simulink model "temp"  (R2013b)
settings: Solver=ode45  StartTime=0.0  StopTime=100*100  RelTol=1e-3
undefined symbols (not defined in the file or in its folder): gray
libraries: xbsIndex_r4 x52, dspsigattribs x9, visionsinks x3, visionsources x1
settings Model: Creator=Sechw  LastModifiedBy=Sechw

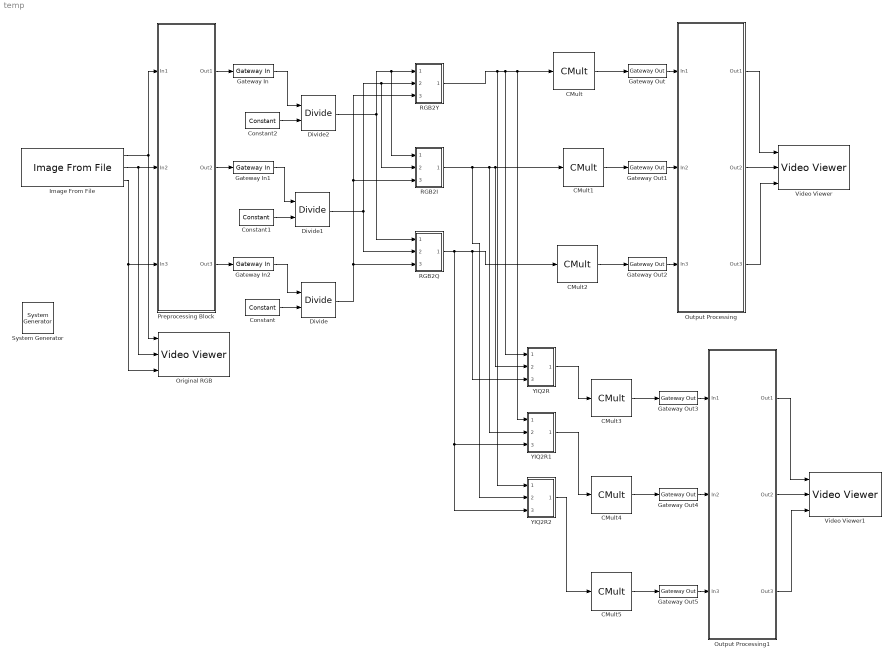
== system temp ==
  " System Generator" : xbsIndex_r4/ System Generator  Tag=genX  xilinxfamily=virtex6  part=xc6vlx130t  speed=-1  package=ff1156  synthesis_tool=XST  clock_wrapper=Clock Enables  directory=./netlist  proj_type=Project Navigator  Synth_file=XST Defaults  Impl_file=ISE Defaults  testbench=off  simulink_period=1  sysclk_period=10  dcm_input_clock_period=10  incr_netlist=off  trim_vbits=Everywhere in SubSystem  dbl_ovrd=According to Block Masks  core_generation=According to Block Masks  run_coregen=off  deprecated_control=off  eval_field=0  block_type=sysgen
  CMult{,1..5} (6 alike) : xbsIndex_r4/CMult  const=255  gui_display_data_type=Floating-point  const_n_bits=16  const_bin_pt=14  float_type=Double  exp_bits=8  fraction_bits=24  en=off  latency=0  precision=Full  arith_type="Signed  (2's comp)"  n_bits=16  bin_pt=14  quantization=Truncate  overflow=Wrap  dbl_ovrd=off  use_behavioral_HDL=off  mem_type=Distributed RAM  pipeline=off  block_type=cmult
  Constant : xbsIndex_r4/Constant  const=255  gui_display_data_type=Floating-point  arith_type=Floating-point  n_bits=16  bin_pt=14  preci_type=Double  exp_width=8  frac_width=24  explicit_period=off  period=1  equ=P=C  opselect=C  inp2=PCIN>>17  opr=+  inp1=P  carry=CIN  dbl_ovrd=off  block_type=constant
  Constant1 : xbsIndex_r4/Constant  const=255  gui_display_data_type=Floating-point  arith_type=Floating-point  n_bits=16  bin_pt=14  preci_type=Double  exp_width=8  frac_width=24  explicit_period=off  period=1  equ=P=C  opselect=C  inp2=PCIN>>17  opr=+  inp1=P  carry=CIN  dbl_ovrd=off  block_type=constant
  Constant2 : xbsIndex_r4/Constant  const=255  gui_display_data_type=Floating-point  arith_type=Floating-point  n_bits=16  bin_pt=14  preci_type=Double  exp_width=8  frac_width=24  explicit_period=off  period=1  equ=P=C  opselect=C  inp2=PCIN>>17  opr=+  inp1=P  carry=CIN  dbl_ovrd=off  block_type=constant
  Divide : xbsIndex_r4/Divide  flow_control=NonBlocking  axi_optimize_goal=Resources  algorithm_type=High_Radix  infoedit1=Specify output fraction-width for Fixed-point division.  fractional_width=16  latency=0  rate=1  has_a_tlast=off  has_a_tuser=off  has_b_tlast=off  has_b_tuser=off  en=off  has_result_tready=off  result_tlast_behv=Pass_A_TLAST  has_underflow=off  has_overflow=off  has_invalid_op=off  has_divide_by_zero=off  fpo_op_type=mergeddivide  block_type=divide
      settings: infoedit=Blocking: Wait for data on all inputs, allow back-pressure.<br>NonBlocking: operate every cycle in which all inputs are valid, no back-pressure.
  Divide1 : xbsIndex_r4/Divide  flow_control=NonBlocking  axi_optimize_goal=Resources  algorithm_type=High_Radix  infoedit1=Specify output fraction-width for Fixed-point division.  fractional_width=16  latency=0  rate=1  has_a_tlast=off  has_a_tuser=off  has_b_tlast=off  has_b_tuser=off  en=off  has_result_tready=off  result_tlast_behv=Pass_A_TLAST  has_underflow=off  has_overflow=off  has_invalid_op=off  has_divide_by_zero=off  fpo_op_type=mergeddivide  block_type=divide
      settings: infoedit=Blocking: Wait for data on all inputs, allow back-pressure.<br>NonBlocking: operate every cycle in which all inputs are valid, no back-pressure.
  Divide2 : xbsIndex_r4/Divide  flow_control=NonBlocking  axi_optimize_goal=Resources  algorithm_type=High_Radix  infoedit1=Specify output fraction-width for Fixed-point division.  fractional_width=16  latency=0  rate=1  has_a_tlast=off  has_a_tuser=off  has_b_tlast=off  has_b_tuser=off  en=off  has_result_tready=off  result_tlast_behv=Pass_A_TLAST  has_underflow=off  has_overflow=off  has_invalid_op=off  has_divide_by_zero=off  fpo_op_type=mergeddivide  block_type=divide
      settings: infoedit=Blocking: Wait for data on all inputs, allow back-pressure.<br>NonBlocking: operate every cycle in which all inputs are valid, no back-pressure.
  Gateway In : xbsIndex_r4/Gateway In  gui_display_data_type=Floating-point  arith_type=Floating-point  n_bits=8  bin_pt=0  preci_type=Double  exp_width=8  frac_width=24  quantization="Round  (unbiased: +/- Inf)"  overflow=Saturate  period=1  dbl_ovrd=off  timing_constraint=None  locs_specified=off  LOCs={}  UseAsADC=off  ADCChannel='1'  inherit_from_input=off  hdl_port=on  block_type=gatewayin
  Gateway In1 : xbsIndex_r4/Gateway In  gui_display_data_type=Floating-point  arith_type=Floating-point  n_bits=8  bin_pt=0  preci_type=Double  exp_width=8  frac_width=24  quantization="Round  (unbiased: +/- Inf)"  overflow=Saturate  period=1  dbl_ovrd=off  timing_constraint=None  locs_specified=off  LOCs={}  UseAsADC=off  ADCChannel='1'  inherit_from_input=off  hdl_port=on  block_type=gatewayin
  Gateway In2 : xbsIndex_r4/Gateway In  gui_display_data_type=Floating-point  arith_type=Floating-point  n_bits=8  bin_pt=0  preci_type=Double  exp_width=8  frac_width=24  quantization="Round  (unbiased: +/- Inf)"  overflow=Saturate  period=1  dbl_ovrd=off  timing_constraint=None  locs_specified=off  LOCs={}  UseAsADC=off  ADCChannel='1'  inherit_from_input=off  hdl_port=on  block_type=gatewayin
  Gateway Out{,1..5} (6 alike) : xbsIndex_r4/Gateway Out  inherit_from_input=on  hdl_port=on  timing_constraint=None  locs_specified=off  LOCs={}  UseAsDAC=off  DACChannel='1'  block_type=gatewayout
  Image From File : visionsources/Image From File  Tag=vipblks_nd  FileName=C:\Users\Sechw\Documents\MATLAB\4440\lena.jpg  imagePorts=Separate color signals  Ts=inf  ImageDataType=Inherit from input image  Signed=on  WordLength=16  sdImageDataType=uint(8)  FractionLengthMode=User-defined  FractionLength=15  OutPortLabels=R|G|B
  Original RGB : visionsinks/Video Viewer  inputType=Obsolete7b  imagePorts=Separate color signals  useColorMap=off  colormapValue=gray(256)  specRange=off  minInputVal=0  maxInputVal=255  FigPos=[692 476 183 243]  AxisZoom=on  trueSizedOnce=off  OpenAtMdlStart=on  DefaultConfigurationName=vipscopes.VideoViewerScopeCfg
  Output Processing : Subsystem
  Output Processing1 : Subsystem
  Preprocessing Block : Subsystem
  RGB2I : Subsystem
  RGB2Q : Subsystem
  RGB2Y : Subsystem
  Video Viewer : visionsinks/Video Viewer  inputType=Obsolete7b  imagePorts=Separate color signals  useColorMap=off  colormapValue=gray(256)  specRange=off  minInputVal=0  maxInputVal=255  FigPos=[437 462 320 274]  AxisZoom=on  trueSizedOnce=off  OpenAtMdlStart=on  DefaultConfigurationName=vipscopes.VideoViewerScopeCfg
  Video Viewer1 : visionsinks/Video Viewer  inputType=Obsolete7b  imagePorts=Separate color signals  useColorMap=off  colormapValue=gray(256)  specRange=off  minInputVal=0  maxInputVal=255  FigPos=[775 461 441 293]  AxisZoom=on  trueSizedOnce=off  OpenAtMdlStart=on  DefaultConfigurationName=vipscopes.VideoViewerScopeCfg
  YIQ2R : Subsystem
  YIQ2R1 : Subsystem
  YIQ2R2 : Subsystem
  wires:
  Image From File/1 -> Preprocessing Block/1(In1), Original RGB/1
  Image From File/2 -> Original RGB/2, Preprocessing Block/2(In2)
  Image From File/3 -> Original RGB/3, Preprocessing Block/3(In3)
  Preprocessing Block/1(Out1) -> Gateway In/1
  Preprocessing Block/2(Out2) -> Gateway In1/1
  Preprocessing Block/3(Out3) -> Gateway In2/1
  Gateway Out/1 -> Output Processing/1(In1)
  Gateway Out1/1 -> Output Processing/2(In2)
  Gateway Out2/1 -> Output Processing/3(In3)
  Output Processing/1(Out1) -> Video Viewer/1
  Output Processing/2(Out2) -> Video Viewer/2
  Output Processing/3(Out3) -> Video Viewer/3
  Divide2/1 -> RGB2I/1(In1), RGB2Y/1(In1), RGB2Q/1(In1)
  Divide1/1 -> RGB2I/2(In2), RGB2Y/2(In2), RGB2Q/2(In2)
  Divide/1 -> RGB2Q/3(In3), RGB2Y/3(In3), RGB2I/3(In3)
  RGB2Y/1(Out1) -> YIQ2R2/1(In1), YIQ2R/1(In1), YIQ2R1/1(In1), CMult/1
  RGB2I/1(Out1) -> YIQ2R2/2(In2), YIQ2R1/2(In2), YIQ2R/2(In2), CMult1/1
  RGB2Q/1(Out1) -> YIQ2R2/3(In3), YIQ2R1/3(In3), YIQ2R/3(In3), CMult2/1
  Gateway Out3/1 -> Output Processing1/1(In1)
  Gateway Out4/1 -> Output Processing1/2(In2)
  Gateway Out5/1 -> Output Processing1/3(In3)
  Output Processing1/1(Out1) -> Video Viewer1/1
  Output Processing1/2(Out2) -> Video Viewer1/2
  Output Processing1/3(Out3) -> Video Viewer1/3
  YIQ2R/1(Out1) -> CMult3/1
  YIQ2R1/1(Out1) -> CMult4/1
  YIQ2R2/1(Out1) -> CMult5/1
  Gateway In2/1 -> Divide/1
  Constant/1 -> Divide/2
  CMult/1 -> Gateway Out/1
  CMult1/1 -> Gateway Out1/1
  CMult2/1 -> Gateway Out2/1
  Gateway In1/1 -> Divide1/1
  Constant1/1 -> Divide1/2
  Gateway In/1 -> Divide2/1
  Constant2/1 -> Divide2/2
  CMult3/1 -> Gateway Out3/1
  CMult4/1 -> Gateway Out4/1
  CMult5/1 -> Gateway Out5/1

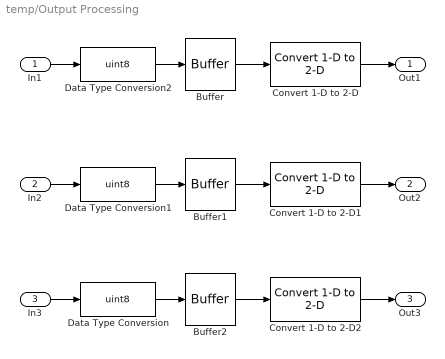
== system temp/Output Processing ==
  In1 : Inport
  In2 : Inport  Port=2
  In3 : Inport  Port=3
  Buffer : Buffer  N=100*100  TreatMby1Signals=One channel
  Buffer1 : Buffer  N=100*100  TreatMby1Signals=One channel
  Buffer2 : Buffer  N=100*100  TreatMby1Signals=One channel
  Convert 1-D to 2-D : dspsigattribs/Convert 1-D to 2-D  M=100  N=100  frameBasedOut=off
  Convert 1-D to 2-D1 : dspsigattribs/Convert 1-D to 2-D  M=100  N=100  frameBasedOut=off
  Convert 1-D to 2-D2 : dspsigattribs/Convert 1-D to 2-D  M=100  N=100  frameBasedOut=off
  Data Type Conversion : DataTypeConversion  OutDataTypeStr=uint8
  Data Type Conversion1 : DataTypeConversion  OutDataTypeStr=uint8
  Data Type Conversion2 : DataTypeConversion  OutDataTypeStr=uint8
  Out1 : Outport
  Out2 : Outport  Port=2
  Out3 : Outport  Port=3
  wires:
  Convert 1-D to 2-D2/1 -> Out3/1
  Convert 1-D to 2-D1/1 -> Out2/1
  Buffer1/1 -> Convert 1-D to 2-D1/1
  Buffer2/1 -> Convert 1-D to 2-D2/1
  Buffer/1 -> Convert 1-D to 2-D/1
  Convert 1-D to 2-D/1 -> Out1/1
  In1/1 -> Data Type Conversion2/1
  In2/1 -> Data Type Conversion1/1
  In3/1 -> Data Type Conversion/1
  Data Type Conversion/1 -> Buffer2/1
  Data Type Conversion1/1 -> Buffer1/1
  Data Type Conversion2/1 -> Buffer/1

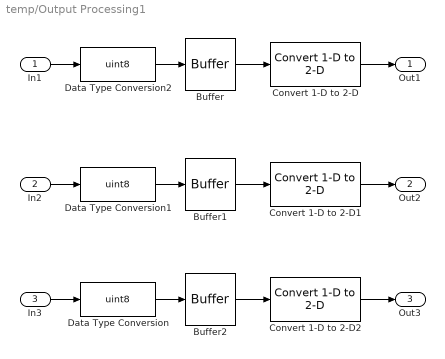
== system temp/Output Processing1 ==
  In1 : Inport
  In2 : Inport  Port=2
  In3 : Inport  Port=3
  Buffer : Buffer  N=100*100  TreatMby1Signals=One channel
  Buffer1 : Buffer  N=100*100  TreatMby1Signals=One channel
  Buffer2 : Buffer  N=100*100  TreatMby1Signals=One channel
  Convert 1-D to 2-D : dspsigattribs/Convert 1-D to 2-D  M=100  N=100  frameBasedOut=off
  Convert 1-D to 2-D1 : dspsigattribs/Convert 1-D to 2-D  M=100  N=100  frameBasedOut=off
  Convert 1-D to 2-D2 : dspsigattribs/Convert 1-D to 2-D  M=100  N=100  frameBasedOut=off
  Data Type Conversion : DataTypeConversion  OutDataTypeStr=uint8
  Data Type Conversion1 : DataTypeConversion  OutDataTypeStr=uint8
  Data Type Conversion2 : DataTypeConversion  OutDataTypeStr=uint8
  Out1 : Outport
  Out2 : Outport  Port=2
  Out3 : Outport  Port=3
  wires:
  Convert 1-D to 2-D2/1 -> Out3/1
  Convert 1-D to 2-D1/1 -> Out2/1
  Buffer1/1 -> Convert 1-D to 2-D1/1
  Buffer2/1 -> Convert 1-D to 2-D2/1
  Buffer/1 -> Convert 1-D to 2-D/1
  Convert 1-D to 2-D/1 -> Out1/1
  In1/1 -> Data Type Conversion2/1
  In2/1 -> Data Type Conversion1/1
  In3/1 -> Data Type Conversion/1
  Data Type Conversion/1 -> Buffer2/1
  Data Type Conversion1/1 -> Buffer1/1
  Data Type Conversion2/1 -> Buffer/1

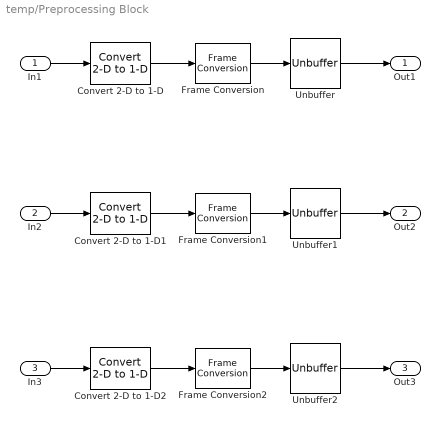
== system temp/Preprocessing Block ==
  In1 : Inport
  In2 : Inport  Port=2
  In3 : Inport  Port=3
  Convert 2-D to 1-D : dspsigattribs/Convert 2-D to 1-D
  Convert 2-D to 1-D1 : dspsigattribs/Convert 2-D to 1-D
  Convert 2-D to 1-D2 : dspsigattribs/Convert 2-D to 1-D
  Frame Conversion : FrameConversion
  Frame Conversion1 : FrameConversion
  Frame Conversion2 : FrameConversion
  Unbuffer : Unbuffer  SampleBasedProcessing=Same as frame based
  Unbuffer1 : Unbuffer  SampleBasedProcessing=Same as frame based
  Unbuffer2 : Unbuffer  SampleBasedProcessing=Same as frame based
  Out1 : Outport
  Out2 : Outport  Port=2
  Out3 : Outport  Port=3
  wires:
  In1/1 -> Convert 2-D to 1-D/1
  Frame Conversion1/1 -> Unbuffer1/1
  Convert 2-D to 1-D1/1 -> Frame Conversion1/1
  In2/1 -> Convert 2-D to 1-D1/1
  Unbuffer1/1 -> Out2/1
  Frame Conversion2/1 -> Unbuffer2/1
  In3/1 -> Convert 2-D to 1-D2/1
  Convert 2-D to 1-D2/1 -> Frame Conversion2/1
  Unbuffer2/1 -> Out3/1
  Unbuffer/1 -> Out1/1
  Frame Conversion/1 -> Unbuffer/1
  Convert 2-D to 1-D/1 -> Frame Conversion/1

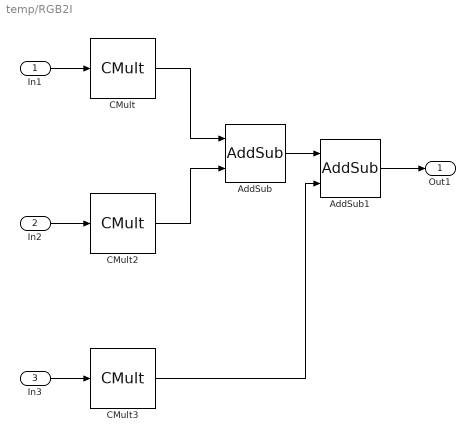
== system temp/RGB2I ==
  In1 : Inport
  In2 : Inport  Port=2
  In3 : Inport  Port=3
  AddSub : xbsIndex_r4/AddSub  mode=Addition  use_carryin=off  use_carryout=off  en=off  latency=0  precision=Full  arith_type=Unsigned  n_bits=16  bin_pt=14  quantization=Truncate  overflow=Wrap  dbl_ovrd=off  use_behavioral_HDL=off  hw_selection=Fabric  pipelined=off  block_type=addsub
  AddSub1 : xbsIndex_r4/AddSub  mode=Addition  use_carryin=off  use_carryout=off  en=off  latency=0  precision=Full  arith_type=Unsigned  n_bits=16  bin_pt=14  quantization=Truncate  overflow=Wrap  dbl_ovrd=off  use_behavioral_HDL=off  hw_selection=Fabric  pipelined=off  block_type=addsub
  CMult : xbsIndex_r4/CMult  const=0.596  gui_display_data_type=Floating-point  const_n_bits=8  const_bin_pt=8  float_type=Double  exp_bits=8  fraction_bits=24  en=off  latency=0  precision=Full  arith_type="Signed  (2's comp)"  n_bits=16  bin_pt=14  quantization=Truncate  overflow=Wrap  dbl_ovrd=off  use_behavioral_HDL=off  mem_type=Distributed RAM  pipeline=off  block_type=cmult
  CMult2 : xbsIndex_r4/CMult  const=-0.275  gui_display_data_type=Floating-point  const_n_bits=8  const_bin_pt=8  float_type=Double  exp_bits=8  fraction_bits=24  en=off  latency=0  precision=Full  arith_type="Signed  (2's comp)"  n_bits=16  bin_pt=14  quantization=Truncate  overflow=Wrap  dbl_ovrd=off  use_behavioral_HDL=off  mem_type=Distributed RAM  pipeline=off  block_type=cmult
  CMult3 : xbsIndex_r4/CMult  const=-0.321  gui_display_data_type=Floating-point  const_n_bits=8  const_bin_pt=8  float_type=Double  exp_bits=8  fraction_bits=24  en=off  latency=0  precision=Full  arith_type="Signed  (2's comp)"  n_bits=16  bin_pt=14  quantization=Truncate  overflow=Wrap  dbl_ovrd=off  use_behavioral_HDL=off  mem_type=Distributed RAM  pipeline=off  block_type=cmult
  Out1 : Outport
  wires:
  In2/1 -> CMult2/1
  CMult2/1 -> AddSub/2
  AddSub/1 -> AddSub1/1
  AddSub1/1 -> Out1/1
  CMult3/1 -> AddSub1/2
  CMult/1 -> AddSub/1
  In3/1 -> CMult3/1
  In1/1 -> CMult/1

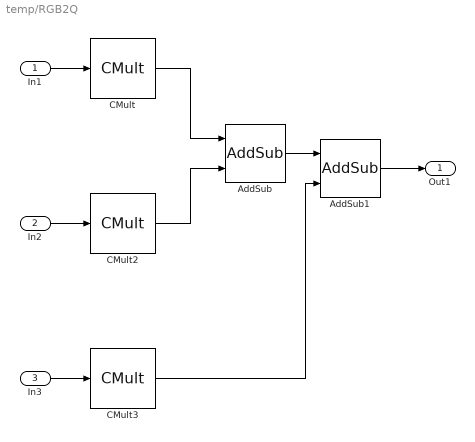
== system temp/RGB2Q ==
  In1 : Inport
  In2 : Inport  Port=2
  In3 : Inport  Port=3
  AddSub : xbsIndex_r4/AddSub  mode=Addition  use_carryin=off  use_carryout=off  en=off  latency=0  precision=Full  arith_type=Unsigned  n_bits=16  bin_pt=14  quantization=Truncate  overflow=Wrap  dbl_ovrd=off  use_behavioral_HDL=off  hw_selection=Fabric  pipelined=off  block_type=addsub
  AddSub1 : xbsIndex_r4/AddSub  mode=Addition  use_carryin=off  use_carryout=off  en=off  latency=0  precision=Full  arith_type=Unsigned  n_bits=16  bin_pt=14  quantization=Truncate  overflow=Wrap  dbl_ovrd=off  use_behavioral_HDL=off  hw_selection=Fabric  pipelined=off  block_type=addsub
  CMult : xbsIndex_r4/CMult  const=0.212  gui_display_data_type=Floating-point  const_n_bits=8  const_bin_pt=8  float_type=Double  exp_bits=8  fraction_bits=24  en=off  latency=0  precision=Full  arith_type="Signed  (2's comp)"  n_bits=16  bin_pt=14  quantization=Truncate  overflow=Wrap  dbl_ovrd=off  use_behavioral_HDL=off  mem_type=Distributed RAM  pipeline=off  block_type=cmult
  CMult2 : xbsIndex_r4/CMult  const=-0.523  gui_display_data_type=Floating-point  const_n_bits=8  const_bin_pt=8  float_type=Double  exp_bits=8  fraction_bits=24  en=off  latency=0  precision=Full  arith_type="Signed  (2's comp)"  n_bits=16  bin_pt=14  quantization=Truncate  overflow=Wrap  dbl_ovrd=off  use_behavioral_HDL=off  mem_type=Distributed RAM  pipeline=off  block_type=cmult
  CMult3 : xbsIndex_r4/CMult  const=0.311  gui_display_data_type=Floating-point  const_n_bits=8  const_bin_pt=8  float_type=Double  exp_bits=8  fraction_bits=24  en=off  latency=0  precision=Full  arith_type="Signed  (2's comp)"  n_bits=16  bin_pt=14  quantization=Truncate  overflow=Wrap  dbl_ovrd=off  use_behavioral_HDL=off  mem_type=Distributed RAM  pipeline=off  block_type=cmult
  Out1 : Outport
  wires:
  In2/1 -> CMult2/1
  CMult2/1 -> AddSub/2
  AddSub/1 -> AddSub1/1
  AddSub1/1 -> Out1/1
  CMult3/1 -> AddSub1/2
  CMult/1 -> AddSub/1
  In3/1 -> CMult3/1
  In1/1 -> CMult/1

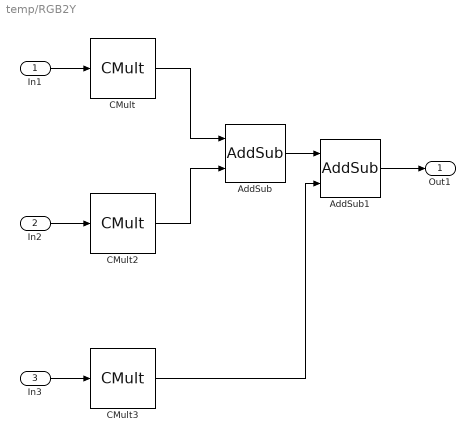
== system temp/RGB2Y ==
  In1 : Inport
  In2 : Inport  Port=2
  In3 : Inport  Port=3
  AddSub : xbsIndex_r4/AddSub  mode=Addition  use_carryin=off  use_carryout=off  en=off  latency=0  precision=Full  arith_type=Unsigned  n_bits=16  bin_pt=14  quantization=Truncate  overflow=Wrap  dbl_ovrd=off  use_behavioral_HDL=off  hw_selection=Fabric  pipelined=off  block_type=addsub
  AddSub1 : xbsIndex_r4/AddSub  mode=Addition  use_carryin=off  use_carryout=off  en=off  latency=0  precision=Full  arith_type=Unsigned  n_bits=16  bin_pt=14  quantization=Truncate  overflow=Wrap  dbl_ovrd=off  use_behavioral_HDL=off  hw_selection=Fabric  pipelined=off  block_type=addsub
  CMult : xbsIndex_r4/CMult  const=0.299  gui_display_data_type=Floating-point  const_n_bits=8  const_bin_pt=8  float_type=Double  exp_bits=8  fraction_bits=24  en=off  latency=0  precision=Full  arith_type="Signed  (2's comp)"  n_bits=16  bin_pt=14  quantization=Truncate  overflow=Wrap  dbl_ovrd=off  use_behavioral_HDL=off  mem_type=Distributed RAM  pipeline=off  block_type=cmult
  CMult2 : xbsIndex_r4/CMult  const=0.587  gui_display_data_type=Floating-point  const_n_bits=8  const_bin_pt=8  float_type=Double  exp_bits=8  fraction_bits=24  en=off  latency=0  precision=Full  arith_type="Signed  (2's comp)"  n_bits=16  bin_pt=14  quantization=Truncate  overflow=Wrap  dbl_ovrd=off  use_behavioral_HDL=off  mem_type=Distributed RAM  pipeline=off  block_type=cmult
  CMult3 : xbsIndex_r4/CMult  const=0.114  gui_display_data_type=Floating-point  const_n_bits=8  const_bin_pt=8  float_type=Double  exp_bits=8  fraction_bits=24  en=off  latency=0  precision=Full  arith_type="Signed  (2's comp)"  n_bits=16  bin_pt=14  quantization=Truncate  overflow=Wrap  dbl_ovrd=off  use_behavioral_HDL=off  mem_type=Distributed RAM  pipeline=off  block_type=cmult
  Out1 : Outport
  wires:
  In2/1 -> CMult2/1
  CMult2/1 -> AddSub/2
  AddSub/1 -> AddSub1/1
  AddSub1/1 -> Out1/1
  CMult3/1 -> AddSub1/2
  CMult/1 -> AddSub/1
  In3/1 -> CMult3/1
  In1/1 -> CMult/1

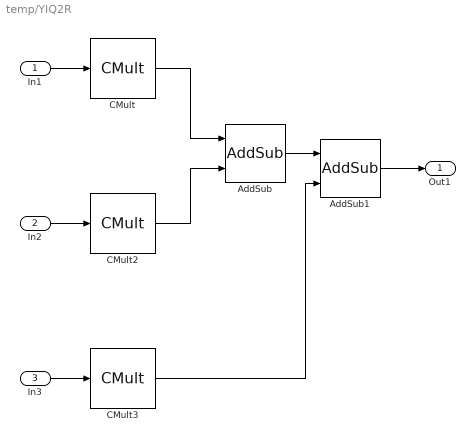
== system temp/YIQ2R ==
  In1 : Inport
  In2 : Inport  Port=2
  In3 : Inport  Port=3
  AddSub : xbsIndex_r4/AddSub  mode=Addition  use_carryin=off  use_carryout=off  en=off  latency=0  precision=Full  arith_type=Unsigned  n_bits=16  bin_pt=14  quantization=Truncate  overflow=Wrap  dbl_ovrd=off  use_behavioral_HDL=off  hw_selection=Fabric  pipelined=off  block_type=addsub
  AddSub1 : xbsIndex_r4/AddSub  mode=Addition  use_carryin=off  use_carryout=off  en=off  latency=0  precision=Full  arith_type=Unsigned  n_bits=16  bin_pt=14  quantization=Truncate  overflow=Wrap  dbl_ovrd=off  use_behavioral_HDL=off  hw_selection=Fabric  pipelined=off  block_type=addsub
  CMult : xbsIndex_r4/CMult  const=1  gui_display_data_type=Floating-point  const_n_bits=8  const_bin_pt=8  float_type=Double  exp_bits=8  fraction_bits=24  en=off  latency=0  precision=Full  arith_type="Signed  (2's comp)"  n_bits=16  bin_pt=14  quantization=Truncate  overflow=Wrap  dbl_ovrd=off  use_behavioral_HDL=off  mem_type=Distributed RAM  pipeline=off  block_type=cmult
  CMult2 : xbsIndex_r4/CMult  const=0.965  gui_display_data_type=Floating-point  const_n_bits=8  const_bin_pt=8  float_type=Double  exp_bits=8  fraction_bits=24  en=off  latency=0  precision=Full  arith_type="Signed  (2's comp)"  n_bits=16  bin_pt=14  quantization=Truncate  overflow=Wrap  dbl_ovrd=off  use_behavioral_HDL=off  mem_type=Distributed RAM  pipeline=off  block_type=cmult
  CMult3 : xbsIndex_r4/CMult  const=0.621  gui_display_data_type=Floating-point  const_n_bits=8  const_bin_pt=8  float_type=Double  exp_bits=8  fraction_bits=24  en=off  latency=0  precision=Full  arith_type="Signed  (2's comp)"  n_bits=16  bin_pt=14  quantization=Truncate  overflow=Wrap  dbl_ovrd=off  use_behavioral_HDL=off  mem_type=Distributed RAM  pipeline=off  block_type=cmult
  Out1 : Outport
  wires:
  In2/1 -> CMult2/1
  CMult2/1 -> AddSub/2
  AddSub/1 -> AddSub1/1
  AddSub1/1 -> Out1/1
  CMult3/1 -> AddSub1/2
  CMult/1 -> AddSub/1
  In3/1 -> CMult3/1
  In1/1 -> CMult/1

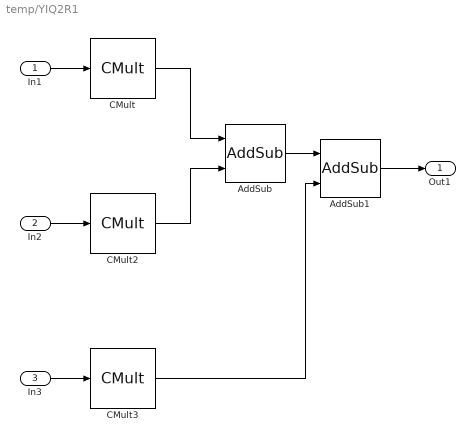
== system temp/YIQ2R1 ==
  In1 : Inport
  In2 : Inport  Port=2
  In3 : Inport  Port=3
  AddSub : xbsIndex_r4/AddSub  mode=Addition  use_carryin=off  use_carryout=off  en=off  latency=0  precision=Full  arith_type=Unsigned  n_bits=16  bin_pt=14  quantization=Truncate  overflow=Wrap  dbl_ovrd=off  use_behavioral_HDL=off  hw_selection=Fabric  pipelined=off  block_type=addsub
  AddSub1 : xbsIndex_r4/AddSub  mode=Addition  use_carryin=off  use_carryout=off  en=off  latency=0  precision=Full  arith_type=Unsigned  n_bits=16  bin_pt=14  quantization=Truncate  overflow=Wrap  dbl_ovrd=off  use_behavioral_HDL=off  hw_selection=Fabric  pipelined=off  block_type=addsub
  CMult : xbsIndex_r4/CMult  const=1  gui_display_data_type=Floating-point  const_n_bits=8  const_bin_pt=8  float_type=Double  exp_bits=8  fraction_bits=24  en=off  latency=0  precision=Full  arith_type="Signed  (2's comp)"  n_bits=16  bin_pt=14  quantization=Truncate  overflow=Wrap  dbl_ovrd=off  use_behavioral_HDL=off  mem_type=Distributed RAM  pipeline=off  block_type=cmult
  CMult2 : xbsIndex_r4/CMult  const=-0.272  gui_display_data_type=Floating-point  const_n_bits=8  const_bin_pt=8  float_type=Double  exp_bits=8  fraction_bits=24  en=off  latency=0  precision=Full  arith_type="Signed  (2's comp)"  n_bits=16  bin_pt=14  quantization=Truncate  overflow=Wrap  dbl_ovrd=off  use_behavioral_HDL=off  mem_type=Distributed RAM  pipeline=off  block_type=cmult
  CMult3 : xbsIndex_r4/CMult  const=-0.647  gui_display_data_type=Floating-point  const_n_bits=8  const_bin_pt=8  float_type=Double  exp_bits=8  fraction_bits=24  en=off  latency=0  precision=Full  arith_type="Signed  (2's comp)"  n_bits=16  bin_pt=14  quantization=Truncate  overflow=Wrap  dbl_ovrd=off  use_behavioral_HDL=off  mem_type=Distributed RAM  pipeline=off  block_type=cmult
  Out1 : Outport
  wires:
  In2/1 -> CMult2/1
  CMult2/1 -> AddSub/2
  AddSub/1 -> AddSub1/1
  AddSub1/1 -> Out1/1
  CMult3/1 -> AddSub1/2
  CMult/1 -> AddSub/1
  In3/1 -> CMult3/1
  In1/1 -> CMult/1

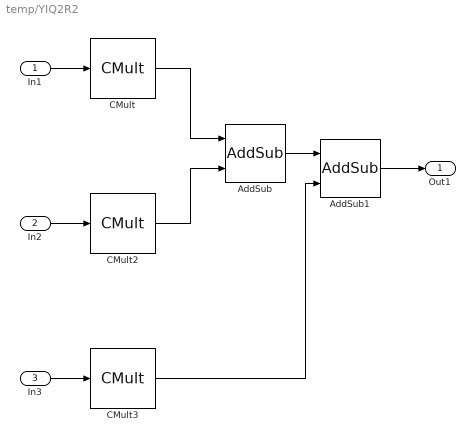
== system temp/YIQ2R2 ==
  In1 : Inport
  In2 : Inport  Port=2
  In3 : Inport  Port=3
  AddSub : xbsIndex_r4/AddSub  mode=Addition  use_carryin=off  use_carryout=off  en=off  latency=0  precision=Full  arith_type=Unsigned  n_bits=16  bin_pt=14  quantization=Truncate  overflow=Wrap  dbl_ovrd=off  use_behavioral_HDL=off  hw_selection=Fabric  pipelined=off  block_type=addsub
  AddSub1 : xbsIndex_r4/AddSub  mode=Addition  use_carryin=off  use_carryout=off  en=off  latency=0  precision=Full  arith_type=Unsigned  n_bits=16  bin_pt=14  quantization=Truncate  overflow=Wrap  dbl_ovrd=off  use_behavioral_HDL=off  hw_selection=Fabric  pipelined=off  block_type=addsub
  CMult : xbsIndex_r4/CMult  const=1  gui_display_data_type=Floating-point  const_n_bits=8  const_bin_pt=8  float_type=Double  exp_bits=8  fraction_bits=24  en=off  latency=0  precision=Full  arith_type="Signed  (2's comp)"  n_bits=16  bin_pt=14  quantization=Truncate  overflow=Wrap  dbl_ovrd=off  use_behavioral_HDL=off  mem_type=Distributed RAM  pipeline=off  block_type=cmult
  CMult2 : xbsIndex_r4/CMult  const=-1.105  gui_display_data_type=Floating-point  const_n_bits=8  const_bin_pt=8  float_type=Double  exp_bits=8  fraction_bits=24  en=off  latency=0  precision=Full  arith_type="Signed  (2's comp)"  n_bits=16  bin_pt=14  quantization=Truncate  overflow=Wrap  dbl_ovrd=off  use_behavioral_HDL=off  mem_type=Distributed RAM  pipeline=off  block_type=cmult
  CMult3 : xbsIndex_r4/CMult  const=1.702  gui_display_data_type=Floating-point  const_n_bits=8  const_bin_pt=8  float_type=Double  exp_bits=8  fraction_bits=24  en=off  latency=0  precision=Full  arith_type="Signed  (2's comp)"  n_bits=16  bin_pt=14  quantization=Truncate  overflow=Wrap  dbl_ovrd=off  use_behavioral_HDL=off  mem_type=Distributed RAM  pipeline=off  block_type=cmult
  Out1 : Outport
  wires:
  In2/1 -> CMult2/1
  CMult2/1 -> AddSub/2
  AddSub/1 -> AddSub1/1
  AddSub1/1 -> Out1/1
  CMult3/1 -> AddSub1/2
  CMult/1 -> AddSub/1
  In3/1 -> CMult3/1
  In1/1 -> CMult/1
